simulink model "MicroFSMPCCLACPU1"  (R2024a)
settings: Solver=FixedStepAuto  StartTime=0.0  StopTime=Inf  RelTol=1e-3  EnableMultiTasking=on
values from neighbouring files (symbols this model uses):
  ar = single(round(1/10,3))    [Para_Motor_Micro.m]
  PI_params = mcb.internal.SetControllerParameters(pmsm,inverter,SI_System,T_pwm,Ts,Ts_speed)    [Para_Motor_Micro.m]
  Tabf = round(Tab',3)    [Para_Motor_Micro.m]
  target = mcb_SetProcessorDetails('F28379D',PWM_frequency)    [Para_Motor_Micro.m]
  Ts = T_pwm    (= 3e-05)    [Para_Motor_Micro.m]
  Ts_com = 2*1*Ts    (= 6e-05)    [Para_Motor_Micro.m]
undefined symbols (not defined in the file or in its folder): C28x, codertarget, CPU1, CPU2, Down, dyV, gmax, GPTRIP1SEL, GPTRIP2SEL, inverter, Ls, PWM_Counter_PeriodVel, R, Tab, Tv, Tvz, TZ1, TZ2, ud, Up
libraries: mcbcontrolslib x28, c2802xlib x18, c2837xDlib x13, dsparch4 x6, eeTransforms x5, slpidlib x4, mcbpositiondecoderlib x3, simulink x2, c2806xlib x1, spsabctoAlphaBetaZeroLib x1, c280xlib x1, c2000lib x1
(part 5 of 8)

== matlab function MicroFSMPCCLACPU1/ADC-PWM /Control_System/Current and BEMF gen Trapezoidal/Current trajectory2 ==
  settings: updateMethod=DISCRETE
  data: torq input; Ia output; th input; Ib output; moder output; eab output; w input
function [Ia,Ib,moder,eab]       = fcn(torq,th,w)

Ip=single(torq);


%%%% wrap

%tre = single((1)*th);
Ke=single(0.3631);
 f = single(2*pi);
 tr =single( mod(th,f));
i_A = single(0); i_B = single(0); 
mode=single(0);
e_A = single(0); e_B = single(0); e_C =single(0);


%%%%%%%%%Hexagono
if(0<=tr && tr<=pi/3)
    i_A = single(-3*tr*sqrt(3)/(2*pi));
     i_B = single(-3*tr/(2*pi) +1);

       elseif(pi/3<tr && tr<2*pi/3)
    i_A = single(-sqrt(3)/(2));
     i_B = single(-3*tr/(pi)+1.5);

       elseif(2*pi/3<tr && tr<pi)
    i_A =single( 3*tr*sqrt(3)/(2*pi)-3*sqrt(3)/(2));
     i_B = single(-3*tr/(2*pi) +1/2);

       elseif(pi<tr && tr<4*pi/3)
    i_A =single( 3*tr*sqrt(3)/(2*pi)-3*sqrt(3)/(2));
     i_B = single(3*tr/(2*pi) -5/2);

        elseif(4*pi/3<tr && tr<5*pi/3)
      i_A = single(sqrt(3)/(2));
     i_B =single( 3*tr/(pi)-4.5);

        elseif(5*pi/3<tr && tr<6*pi/3)
          i_A =single( -3*tr*sqrt(3)/(2*pi)+3*sqrt(3));
     i_B = single(3*tr/(2*pi) -2);
 
else
         i_A = single(0);
end



%%%%%%%%%FCEM%%%%%%%%%%%%
%% e_A
if(0<=tr && tr<=pi/6)
    e_A = single(6*tr/pi);
elseif((pi)/6<tr && tr<=5*pi/6)
    e_A = single(1);
  elseif(5*pi/6<tr && tr<=(7*pi)/6)
        e_A = single(-6*(tr-pi)/pi);
    elseif((7*pi)/6<tr && tr<11*pi/6)
        e_A = single(-1);
          elseif((11*pi)/6<tr && tr<12*pi/6)
        e_A =single(6*(tr-2*pi)/pi);
end
%% e_B
if(0<=tr && tr<=pi/2)
    e_B = single(-1);
elseif(pi/2<tr && tr<=(5*pi)/6)
    e_B =single( 6*(tr-4*pi/6)/pi);
elseif((5*pi)/6<tr && tr<=(3*pi)/2)
    e_B = single(1);
  elseif((3*pi)/2<tr && tr<=(11*pi)/6)
        e_B = single(-6*(tr-10*pi/6)/pi);
    elseif((11*pi)/6<tr && tr<2*pi)
        e_B = single(-1);
end
%% e_C
if(0<=tr && tr<=pi/6)
    e_C = single(1);
elseif(pi/6<tr && tr<=(pi)/2)
    e_C = single(-6*(tr-2*pi/6)/pi);
elseif((pi)/2<tr && tr<=(7*pi)/6)
    e_C = single(-1);
  elseif((7*pi)/6<tr && tr<=(3*pi)/2)
        e_C = single(6*(tr-8*pi/6)/pi);
    elseif((3*pi)/2<tr && tr<2*pi)
        e_C = single(1);
end



%%%%%
era=single(Ke*w*e_A);
erb=single(Ke*w*e_B);
erc=single(Ke*w*e_C);
%Ia=Ira;
ea=single((2/3)*(era-(1/2)*(erb)-(1/2)*erc));
eb=single((2/3)*((sqrt(3)/2)*(erb)-(sqrt(3)/2)*erc));

eab=[ea;eb];

%%%%%%%%%%%%%%%%%%%%%%%%

%%%%%%%%Moder%%%%%%%%%%%
if(0<=tr && tr<pi/6)
    mode=single(2);
elseif(pi/6<=tr && tr<(3*pi)/6)
      mode=single(3);
elseif((3*pi)/6<=tr && tr<(5*pi)/6)
    mode=single(4);
  elseif((5*pi)/6<=tr && tr<(7*pi)/6)
          mode=single(5);
    elseif((7*pi)/6<=tr && tr<(9*pi)/6)
         mode=single(6);     
    elseif((9*pi)/6<=tr && tr<(11*pi)/6)
        mode=single(1);
        elseif((11*pi)/6<=tr && tr<(12*pi)/6)
        mode=single(2);
end



moder=single(mode);
%%%%%%%%%%%%%%%%%%


Ia=Ip*2/sqrt(3)*i_A;
Ib=Ip*2/sqrt(3)*i_B;

%%%%%

== matlab function MicroFSMPCCLACPU1/ADC-PWM /Mesurments/Voltage Mesurment/Pole to phase 1 ==
  data: Vag input; Vn output; Vbg input; Vcg input

function Vn  = fcn(Vag,Vbg,Vcg)
% Vg=[Vag;Vbg;Vcg];
% Vn=[2/3,-1/3,-1/3;-1/3,2/3,-1/3;-1/3,-1/3,2/3]*Vg;
% 
 Van=single(2/3*Vag-1/3*Vbg -1/3*Vcg) ;
 Vbn=single(2/3*Vbg-1/3*Vag -1/3*Vcg) ;
 Vcn=single(2/3*Vcg-1/3*Vbg -1/3*Vag) ;
Vn=[Van;Vbn;Vcn];
end

== matlab function MicroFSMPCCLACPU1/ADC-PWM /Control_System/Current and BEMF gen Sinusoidal/Current trajectory1 ==
  settings: updateMethod=DISCRETE
  data: torq input; Ip output; th input; tr output; moder output
function [Ip,tr,moder]       = fcn(torq,th)
%Kt =0.3811;
%Kt=0.3455;
%J= 0.0002618;

%Ke=0.3739;
%Ke=single(0.3631);
%J=single(2.3998e-4);%%%Solo motor
%Ip=single((torq)/(2*Ke));
Ip=single((torq));
% the = (8/2)*th ;
 f = single(2*pi);
 tr =single( mod(th,f));
%tr = single((1)*th);

mode=single(0);


if(0<=tr && tr<pi/6)
    mode=single(2);
elseif(pi/6<=tr && tr<(3*pi)/6)
      mode=single(3);
elseif((3*pi)/6<=tr && tr<(5*pi)/6)
    mode=single(4);
  elseif((5*pi)/6<=tr && tr<(7*pi)/6)
          mode=single(5);
    elseif((7*pi)/6<=tr && tr<(9*pi)/6)
         mode=single(6);     
    elseif((9*pi)/6<=tr && tr<(11*pi)/6)
        mode=single(1);
        elseif((11*pi)/6<=tr && tr<(12*pi)/6)
        mode=single(2);
end




moder=single(mode);

== matlab function MicroFSMPCCLACPU1/ADC-PWM /Control_System/Closed Loop Control/Calculo directo BFEM1 ==
  settings: updateMethod=DISCRETE
  data: Iab input; u input; Iant input; FCEM output size=2
function FCEM     = fcn(Iab,u,Iant)

Ts=single(5e-05);
% R=single(1) ;
% L=single(2.002e-3);
R=single(1) ;
%L=single(9.75e-3);
 L=single(2.1e-3);
%M=(3/7)*L;
%Lt=(7/3)*M;
%Ls=single(L+M);
Ls=single(L);



ea=u(1)-(Ls/Ts)*Iab(1)-(R-(Ls/Ts))*Iant(1);
eb=u(2)-(Ls/Ts)*Iab(2)-(R-(Ls/Ts))*Iant(2);



FCEM=[ea;eb];

== matlab function MicroFSMPCCLACPU1/ADC-PWM /Control_System/Closed Loop Control/Clark Transform Filter/Calculo BEMF ==
  settings: updateMethod=DISCRETE
  data: I input; Iab output
function Iab            = fcn(I)



IA=I(1);
IB=I(2);
IC=I(3);

Ia=single((2/3)*(IA-(1/2)*(IB)-(1/2)*IC));
Ib=single((2/3)*((sqrt(3)/2)*(IB)-(sqrt(3)/2)*IC));

Iab=[Ia;Ib];





%%%%%

== matlab function MicroFSMPCCLACPU1/ADC-PWM /Control_System/CLA Subsystem Current control/Calculo directo BFEM1 ==
  settings: updateMethod=DISCRETE
  data: Iab input; u input; Iant input; FCEM output size=2
function FCEM     = fcn(Iab,u,Iant)

Ts=single(5e-05);
% R=single(1) ;
% L=single(2.002e-3);
R=single(1) ;
%L=single(9.75e-3);
 L=single(2.1e-3);
%M=(3/7)*L;
%Lt=(7/3)*M;
%Ls=single(L+M);
Ls=single(L);



ea=u(1)-(Ls/Ts)*Iab(1)-(R-(Ls/Ts))*Iant(1);
eb=u(2)-(Ls/Ts)*Iab(2)-(R-(Ls/Ts))*Iant(2);



FCEM=[ea;eb];

== matlab function MicroFSMPCCLACPU1/ADC-PWM /Control_System/Closed Loop Control/Current trajectory1 ==
  settings: updateMethod=DISCRETE
  data: torq input; Ia output; th input; Ib output; moder output
function [Ia,Ib,moder]       = fcn(torq,th)
%Kt =0.3811;
%Kt=0.3455;
%J= 0.0002618;
%Ip=single((torq)/(2*Kt));
Ip=single(torq);
% p=single(8);
% Am =single( (6/pi));
% mph = single(pi/3);
%%%% wrap
tr = single((1)*th);
 %f = single(2*pi);
%tr =single( mod(the,f));
i_A = single(0); i_B = single(0); i_C =single(0);
mode=single(0);


%%%%%%%%%Hexagono
% if(0<=tr && tr<=pi/3)
%     i_A = single(0);
%      i_B = single(2/(sqrt(3)));
% 
%        elseif(pi/3<tr && tr<2*pi/3)
%     i_A = single(-1);
%      i_B = single(1/(sqrt(3)));
% 
%        elseif(2*pi/3<tr && tr<pi)
%     i_A =single(-1);
%      i_B = single(-1/(sqrt(3)));
% 
%        elseif(pi<tr && tr<4*pi/3)
%     i_A =single(0);
%      i_B = single(-2/(sqrt(3)));
% 
%         elseif(4*pi/3<tr && tr<5*pi/3)
%       i_A = single(1);
%      i_B =single( -1/(sqrt(3)));
% 
%         elseif(5*pi/3<tr && tr<6*pi/3)
%           i_A =single( 1);
%      i_B = single(3*tr/(2*pi) -2);
%  
% else
%          i_A = single(0);
% end


%%%%%%%%%%%%%%%%%%
if(0<=tr && tr<pi/6)
    mode=single(2);
      i_A = single(0);
     i_B = single(2/(sqrt(3)));

elseif(pi/6<=tr && tr<(3*pi)/6)
      mode=single(3);
         i_A = single(-1);
     i_B = single(1/(sqrt(3)));

elseif((3*pi)/6<=tr && tr<(5*pi)/6)
    mode=single(4);
    i_A =single(-1);
     i_B = single(-1/(sqrt(3)));

  elseif((5*pi)/6<=tr && tr<(7*pi)/6)
          mode=single(5);
              i_A =single(0);
     i_B = single(-2/(sqrt(3)));

    elseif((7*pi)/6<=tr && tr<(9*pi)/6)
         mode=single(6);     
            i_A =single(1);
            i_B = single(-1/(sqrt(3)));
  
    elseif((9*pi)/6<=tr && tr<(11*pi)/6)
        mode=single(1);
                i_A =single( 1);
     i_B = single(1/(sqrt(3)));
        elseif((11*pi)/6<=tr && tr<(12*pi)/6)
        mode=single(2);
     i_A = single(0);
     i_B = single(2/(sqrt(3)));
end
moder=single(mode);



Ia=Ip*i_A;
Ib=Ip*i_B;

%%%%%

== matlab function MicroFSMPCCLACPU1/ADC-PWM /Control_System/Closed Loop Control/Current trajectory12 ==
  settings: updateMethod=DISCRETE
  data: torq input; Ia output; th input; Ib output; mod12 output single size=1; mod6 output single size=1
function [Ia,Ib,mod12,mod6]       = fcn(torq,th)
%Kt =0.3811;
%Kt=0.3455;
%J= 0.0002618;
%Ip=single((torq)/(2*Kt));
Ip=single(torq);
% p=single(8);
% Am =single( (6/pi));
% mph = single(pi/3);
%%%% wrap
tr = single((1)*th);
 %f = single(2*pi);
%tr =single( mod(the,f));
i_A = single(0); i_B = single(0); i_C =single(0);
mode1=single(0);
mode=single(0);

%%%% e_A

if(0<=tr && tr<=pi/6)
    i_A = single(0);
elseif((pi)/6<tr && tr<=5*pi/6)
    i_A = single(-1);
  elseif(5*pi/6<tr && tr<=(7*pi)/6)
        i_A =single( 0);
    elseif((7*pi)/6<tr && tr<11*pi/6)
        i_A = single(1);
          elseif((11*pi)/6<tr && tr<12*pi/6)
        i_A =single(0);
end
%%%% i_B
if(0<=tr && tr<=pi/2)
    i_B = single(1);
elseif(pi/2<tr && tr<=(5*pi)/6)
    i_B = single(0);
elseif((5*pi)/6<tr && tr<=(3*pi)/2)
    i_B = single(-1);
  elseif((3*pi)/2<tr && tr<=(11*pi)/6)
        i_B =single(0);
    elseif((11*pi)/6<tr && tr<2*pi)
        i_B = single(1);
end
%%%% i_C
if(0<=tr && tr<=pi/6)
    i_C = single(-1);
elseif(pi/6<tr && tr<=(pi)/2)
    i_C =single( 0);
elseif((pi)/2<tr && tr<=(7*pi)/6)
    i_C = single(1);
  elseif((7*pi)/6<tr && tr<=(3*pi)/2)
        i_C = single(0);
    elseif((3*pi)/2<tr && tr<2*pi)
        i_C = single(-1);
end
%%%mode
% 
% if(0<=tr && tr<pi/3)
%     mode=1;
% elseif(pi/3<=tr && tr<(2*pi)/3)
%       mode=2;
% elseif((2*pi)/3<=tr && tr<pi)
%     mode=3;
%   elseif(pi<=tr && tr<(4*pi)/3)
%           mode=4;
%     elseif((4*pi)/3<=tr && tr<(5*pi)/3)
%          mode=5;     
%     elseif((5*pi)/3<=tr && tr<2*pi)
%         mode=6;
% end
% 

% if(0<=tr && tr<pi/3)
%     mode=single(1);
% elseif(pi/3<=tr && tr<(2*pi)/3)
%       mode=single(2);
% elseif((2*pi)/3<=tr && tr<pi)
%     mode=single(3);
%   elseif(pi<=tr && tr<(4*pi)/3)
%           mode=single(4);
%     elseif((4*pi)/3<=tr && tr<(5*pi)/3)
%          mode=single(5);     
%     elseif((5*pi)/3<=tr && tr<(6*pi)/3)
%         mode=single(6);
%  end
% moder=single(mode);


% if(0<=tr && tr<pi/6)
%     mode1=single(2);
% elseif(pi/6<=tr && tr<(3*pi)/6)
%       mode1=single(3);
% elseif((3*pi)/6<=tr && tr<(5*pi)/6)
%     mode1=single(4);
%   elseif((5*pi)/6<=tr && tr<(7*pi)/6)
%           mode1=single(5);
%     elseif((7*pi)/6<=tr && tr<(9*pi)/6)
%          mode1=single(6);     
%     elseif((9*pi)/6<=tr && tr<(11*pi)/6)
%         mode1=single(1);
%         elseif((11*pi)/6<=tr && tr<(12*pi)/6)
%         mode1=single(2);
% end



% %%%%12%%%
if(0<=tr && tr<pi/6)
    mode=single(4);
    mode1=single(2);
elseif(pi/6<=tr && tr<(2*pi)/6)
      mode=single(5);
         mode1=single(3);
elseif(2*pi/6<=tr && tr<(3*pi)/6)
      mode=single(6);
         mode1=single(3);
elseif((3*pi)/6<=tr && tr<(4*pi)/6)
    mode=single(7);
    mode1=single(4);
elseif((4*pi)/6<=tr && tr<(5*pi)/6)
    mode=single(8); 
     mode1=single(4);
 elseif((5*pi)/6<=tr && tr<(6*pi)/6)
          mode=single(9);
           mode1=single(5);
 elseif((6*pi)/6<=tr && tr<(7*pi)/6)
          mode=single(10);   
                   mode1=single(5);
    elseif((7*pi)/6<=tr && tr<(8*pi)/6)
         mode=single(11); 
                  mode1=single(6);
  elseif((8*pi)/6<=tr && tr<(9*pi)/6)
         mode=single(12);      
          mode1=single(6);
    elseif((9*pi)/6<=tr && tr<(10*pi)/6)
        mode=single(1);
         mode1=single(1);
    elseif((10*pi)/6<=tr && tr<(11*pi)/6)
        mode=single(2);
            mode1=single(1);
        elseif((11*pi)/6<=tr && tr<(12*pi)/6)
        mode=single(3);
        mode1=single(2);
end

%%%%%



mod6=single(mode1);
mod12=single(mode);
%%%%%
Ira=single(Ip*i_A);
Irb=single(Ip*i_B);
Irc=single(Ip*i_C);
%Ia=Ira;
Ia=single((2/3)*(Ira-(1/2)*(Irb)-(1/2)*Irc));
Ib=single((2/3)*((sqrt(3)/2)*(Irb)-(sqrt(3)/2)*Irc));

%%%%%

== matlab function MicroFSMPCCLACPU1/ADC-PWM /Control_System/Closed Loop Control/Current trayectory moder12 ==
  settings: updateMethod=DISCRETE
  data: torq input; Ia output; th input; Ib output; selector output; moder output
function [Ia,Ib,selector,moder]       = fcn(torq,th)
%Kt =0.3811;
% Kt=0.3739;
% J= 2.9795e-04;
%Ip=(J*torq)/(2*Kt);
Ip=single(torq);
p=single(8);
Am =single( (6/pi));
mph = single(pi/3);
%%%% wrap
tr = single((1)*th);
%tr2 = mod(the,f);
trb=tr-(2*pi)/3;
if (trb<0)
  trb=trb+2*pi;  
end
trc=tr-(4*pi)/3;
if (trc<0)
  trc=trc+2*pi;  
end
i_A =single( 0); i_B = single( 0); i_C = single( 0);
mode=single(0);
mode1=single(0);
%%%% e_A
%%%%%%Hexagono%%%%%
if(0<=tr && tr<=pi/3)
    i_A = single(-3*tr*sqrt(3)/(2*pi));
     i_B = single(-3*tr/(2*pi) +1);

       elseif(pi/3<tr && tr<2*pi/3)
    i_A = single(-sqrt(3)/(2));
     i_B = single(-3*tr/(pi)+1.5);

       elseif(2*pi/3<tr && tr<pi)
    i_A = single(3*tr*sqrt(3)/(2*pi)-3*sqrt(3)/(2));
     i_B = single(-3*tr/(2*pi) +1/2);

       elseif(pi<tr && tr<4*pi/3)
    i_A =single( 3*tr*sqrt(3)/(2*pi)-3*sqrt(3)/(2));
     i_B =single( 3*tr/(2*pi) -5/2);

        elseif(4*pi/3<tr && tr<5*pi/3)
      i_A =single( sqrt(3)/(2));
     i_B = single(3*tr/(pi)-4.5);

        elseif(5*pi/3<tr && tr<6*pi/3)
          i_A =single( -3*tr*sqrt(3)/(2*pi)+3*sqrt(3));
     i_B = single(3*tr/(2*pi) -2);
 
else
         i_A = single(0);
end
%%%%%%%%%%%%%%%%%%%%%%%
%%%%%%%Normal
%%%% e_A

% if(0<=tr && tr<=pi/6)
%     i_A =0;
% elseif((pi)/6<tr && tr<=5*pi/6)
%     i_A = -1;
%   elseif(5*pi/6<tr && tr<=(7*pi)/6)
%         i_A =0;
%     elseif((7*pi)/6<tr && tr<11*pi/6)
%         i_A = 1;
%           elseif((11*pi)/6<tr && tr<12*pi/6)
%         i_A =0;
% end
% %%%% i_B
% if(0<=tr && tr<=pi/2)
%     i_B = 1;
% elseif(pi/2<tr && tr<=(5*pi)/6)
%     i_B = 0;
% elseif((5*pi)/6<tr && tr<=(3*pi)/2)
%     i_B = -1;
%   elseif((3*pi)/2<tr && tr<=(11*pi)/6)
%         i_B =0;
%     elseif((11*pi)/6<tr && tr<2*pi)
%         i_B = 1;
% end
% %%%% i_C
% if(0<=tr && tr<=pi/6)
%     i_C = -1;
% elseif(pi/6<tr && tr<=(pi)/2)
%     i_C =0;
% elseif((pi)/2<tr && tr<=(7*pi)/6)
%     i_C = 1;
%   elseif((7*pi)/6<tr && tr<=(3*pi)/2)
%         i_C = 0;
%     elseif((3*pi)/2<tr && tr<2*pi)
%         i_C = -1;
% end
%%%%%%%%%%

%%%mode
% 
% if(0<=tr && tr<pi/3)
%     mode=1;
% elseif(pi/3<=tr && tr<(2*pi)/3)
%       mode=2;
% elseif((2*pi)/3<=tr && tr<pi)
%     mode=3;
%   elseif(pi<=tr && tr<(4*pi)/3)
%           mode=4;
%     elseif((4*pi)/3<=tr && tr<(5*pi)/3)
%          mode=5;     
%     elseif((5*pi)/3<=tr && tr<2*pi)
%         mode=6;
% end
% 
% if(0<=tr && tr<pi/6)
%     mode=2;
% elseif(pi/6<=tr && tr<(3*pi)/6)
%       mode=3;
% elseif((3*pi)/6<=tr && tr<(5*pi)/6)
%     mode=4;
%   elseif((5*pi)/6<=tr && tr<(7*pi)/6)
%           mode=5;
%     elseif((7*pi)/6<=tr && tr<(9*pi)/6)
%          mode=6;     
%     elseif((9*pi)/6<=tr && tr<(11*pi)/6)
%         mode=1;
%         elseif((11*pi)/6<=tr && tr<(12*pi)/6)
%         mode=2;
% end
% moder=mode;

if(0<=tr && tr<pi/6)
    mode1=single(2);
elseif(pi/6<=tr && tr<(3*pi)/6)
      mode1=single(3);
elseif((3*pi)/6<=tr && tr<(5*pi)/6)
    mode1=single(4);
  elseif((5*pi)/6<=tr && tr<(7*pi)/6)
          mode1=single(5);
    elseif((7*pi)/6<=tr && tr<(9*pi)/6)
         mode1=single(6);     
    elseif((9*pi)/6<=tr && tr<(11*pi)/6)
        mode1=single(1);
        elseif((11*pi)/6<=tr && tr<(12*pi)/6)
        mode1=single(2);
end


%%%%24%%%
% if(0<=tr && tr<pi/12)
%     mode=7;
%     elseif(pi/12<=tr && tr<(2*pi)/12)
%       mode=8;
%      elseif(2*pi/12<=tr && tr<(3*pi)/12)
%       mode=9;
%      elseif(3*pi/12<=tr && tr<(4*pi)/12)
%       mode=10;
%         elseif(4*pi/12<=tr && tr<(5*pi)/12)
%       mode=11;
%         elseif(5*pi/12<=tr && tr<(6*pi)/12)
%       mode=12;
%         elseif(6*pi/12<=tr && tr<(7*pi)/12)
%       mode=13;
%         elseif(7*pi/12<=tr && tr<(8*pi)/12)
%       mode=14;
%         elseif(8*pi/12<=tr && tr<(9*pi)/12)
%       mode=15;
%          elseif(9*pi/12<=tr && tr<(10*pi)/12)
%       mode=16;
%            elseif(10*pi/12<=tr && tr<(11*pi)/12)
%       mode=17;
%            elseif(11*pi/12<=tr && tr<(12*pi)/12)
%       mode=18;
%            elseif(12*pi/12<=tr && tr<(13*pi)/12)
%       mode=19;
%            elseif(13*pi/12<=tr && tr<(14*pi)/12)
%       mode=20;
%            elseif(14*pi/12<=tr && tr<(15*pi)/12)
%       mode=21;
%            elseif(15*pi/12<=tr && tr<(16*pi)/12)
%       mode=22;
%            elseif(16*pi/12<=tr && tr<(17*pi)/12)
%       mode=23;
%            elseif(17*pi/12<=tr && tr<(18*pi)/12)
%       mode=24;  
%        
%           elseif((9*pi)/6<=tr && tr<(19*pi)/12)
%         mode=1;
%     elseif((19*pi)/12<=tr && tr<(20*pi)/12)
%         mode=2;
%         elseif((20*pi)/12<=tr && tr<(21*pi)/12)
%         mode=3;
%          elseif((21*pi)/12<=tr && tr<(22*pi)/12)
%         mode=4;
%           elseif((22*pi)/12<=tr && tr<(23*pi)/12)
%         mode=5;
%             elseif((23*pi)/12<=tr && tr<(24*pi)/12)
%         mode=6;
% end

%%%%%




% %%%%12%%%
if(0<=tr && tr<pi/6)
    mode=single(4);
elseif(pi/6<=tr && tr<(2*pi)/6)
      mode=single(5);
elseif(2*pi/6<=tr && tr<(3*pi)/6)
      mode=single(6);
elseif((3*pi)/6<=tr && tr<(4*pi)/6)
    mode=single(7);
elseif((4*pi)/6<=tr && tr<(5*pi)/6)
    mode=single(8);    
 elseif((5*pi)/6<=tr && tr<(6*pi)/6)
          mode=single(9);
 elseif((6*pi)/6<=tr && tr<(7*pi)/6)
          mode=single(10);        
    elseif((7*pi)/6<=tr && tr<(8*pi)/6)
         mode=single(11); 
  elseif((8*pi)/6<=tr && tr<(9*pi)/6)
         mode=single(12);         
    elseif((9*pi)/6<=tr && tr<(10*pi)/6)
        mode=single(1);
    elseif((10*pi)/6<=tr && tr<(11*pi)/6)
        mode=single(2);
        elseif((11*pi)/6<=tr && tr<(12*pi)/6)
        mode=single(3);
end

%%%%%


 moder=mode1;
 selector=mode;
%%%%%
Ira=Ip*i_A;
Irb=Ip*i_B;
Irc=Ip*i_C;
%Ia=Ira;
% Ia=(2/3)*(Ira-(1/2)*(Irb)-(1/2)*Irc);
% Ib=(2/3)*((sqrt(3)/2)*(Irb)-(sqrt(3)/2)*Irc);
Ia=Ip*2/sqrt(3)*i_A;
Ib=Ip*2/sqrt(3)*i_B;
%%%%%

== matlab function MicroFSMPCCLACPU1/ADC-PWM /Control_System/Closed Loop Control/FS-MPC 2 Vectores correcion moder ==
  settings: updateMethod=DISCRETE
  data: I input; Gate output size=3; FEM input; iAref input; iBref input; J output size=1; Vbus input; Vpred output; mode input; Ipred output

function [Gate,J,Vpred,Ipred]      = fcn(I,FEM,iAref,iBref,Vbus,mode)


%%%%%Init Parameters%%%%%%%
Ts=single(5e-5);
R=single(1.2) ;
L=single(4.75e-3);
M=L;
Lt=(7/3)*M;
Ls=single(Lt+M);
%ud=240;
ud=single(170);
Kt =single(0.3811);
%T0=Ts*(1);
Ke=single(0.3455);
gmax=single(100000);
n=single(3);
Tp=single(Ts*0.9);
uAnull=single(0);
uBnull=single(0);
 persistent    Gop jop Gates iApred iBpred %status1 %tick status1 
     if isempty(Gates)
        Gates=[0,0,0]';
        Gop=gmax;
        jop=single(1);
        iApred=single(0);
        iBpred=single(0);
% status1=[0,0,0;
%  1,0,0	;
% 1,1,0;]; 
     end


%%%%%%Read mesurments%%%%%%%%%%%%
iA=I(1);
iB=I(2);
eA=FEM(1);
eB=FEM(2);
% eA1=FEM1(1);
% eB1=FEM1(2);
% fa=eA/(Ke*w);
% fb=eB/(Ke*w);
% fa1=fa;
% fb1=fb;
% ua=u(1);
% ub=u(2);



 % % %%%7 vectores ordenados ab separados flotando
%  status1=[0,1,0,1,0,1	;
%      1,0,0,0,0,1	;
%  0,0,1,0,0,1	;
%  0,1,1,0,0,0	;
%  0,1,0,0,1,0	;
%  0,0,0,1,1,0	;
%  1,0,0,1,0,0	;];
% 
%  u1=ud*[0	,	0	;
%      1/2	,	sqrt(3)/6 	;
% 0	,	sqrt(3)/3	;
% -1/2	,	sqrt(3)/6 	;
% -1/2	,	-sqrt(3)/6 	;
% 0	,	-sqrt(3)/3	;
% 1/2	,	-sqrt(3)/6 	;
% ];

%%%%%%For loop 3%%%%%%      
% %%%7 vectores ordenados ab tradicionales
%  status1=[1,1,1;
%           1,0,0	;
%           1,1,0;
%           0,1,0;
%            0,1,1	;
%            0,0,1	;
%            1,0,1;
%            ];
% % 
%  u1=ud*[0	,	0	;
%       2/3	,	0	;
%       1/3	,	1/sqrt(3)	;%parece estar aml el vector
%   -1/3	,	1/sqrt(3)	;
%  -2/3	,	0	;
%  -1/3	,	-1/sqrt(3)	;
%   1/3	,	-1/sqrt(3)	;
%   ];

%%%%%Modos 2 vectores con VO

 if mode==1
 status1=[0,0,0;
 1,0,0	;
1,1,0;];   
 u1=ud*[0	,	0	;
2/3	,	0	;
1/3	,	1/sqrt(3)];
elseif mode==2
 status1=[0,0,0;
1,1,0	;
0,1,0	;];   
 u1=ud*[0	,	0	;
1/3	,	1/sqrt(3)	;
-1/3	,	1/sqrt(3)	;];   
elseif mode==3
 status1=[0,0,0;
0,1,0	;
0,1,1	;];   
 u1=ud*[0	,	0	;
-1/3	,	1/sqrt(3)	;
-2/3	,	0	;];  
 elseif mode==4
 status1=[0,0,0;
 0,1,1	;
0,0,1	;];   
 u1=ud*[0	,	0	;
-2/3	,	0	;
-1/3	,	-1/sqrt(3)	;];
 elseif mode==5
 status1=[0,0,0;
 0,0,1	;
1,0,1	;];   
 u1=ud*[0	,	0	;
-1/3	,	-1/sqrt(3)	;
1/3	,	-1/sqrt(3)	;];
 elseif mode==6
 status1=[0,0,0
1,0,1	;
 1,0,0	;];   
 u1=ud*[0	,	0	;
1/3	,	-1/sqrt(3)	;
2/3	,	0	;];

else
 status1=[0,0,0;
 1,0,0	;
1,1,0;];   
 u1=ud*[0	,	0	;
2/3	,	0	;
1/3	,	1/sqrt(3)]; 
end


%%%%%%%%FSMPC%%%%%%%%%%%%%%%%%%%%%%%%%%%%%%%%%%%%%

     Gop=gmax;
      jop=single(1);

%%%%%%For n loop  %%%%%% 
     for j= 1:n    
     uA1=u1(j,1);
     uB1=u1(j,2);

     iA1= iA + (1/Ls)*(Tp*uA1)- (Ts/Ls)*(eA+R*iA);
     iB1=iB + (1/Ls)*(Tp*uB1)- (Ts/Ls)*(eB+R*iB);
     
     G=abs(iAref-iA1)+abs(iBref-iB1) ; 

          if G<Gop
          Gop=G;
          jop=j;
          iApred=iA1;
          iBpred=iB1;
          end
     end

    
%%%%Apply conmutation states%%%%%%%%%%%%%%%%%%%%%%%  

    Gates=status1(jop,:)';
UA=Tp/Ts*u1(jop,1) ;%+(Ts-Tp)/Ts*uAnull;
UB=Tp/Ts*u1(jop,2) ;%+(Ts-Tp)/Ts*uBnull;
%Gates=status1(jop,:)';
J=jop;
Gate=Gates;
Vpred=[UA;UB];
Ipred=[iApred;iBpred];
%tie=t2;
%jl=jn;
%j=1;

== matlab function MicroFSMPCCLACPU1/ADC-PWM /Control_System/Closed Loop Control/FS-MPC 2 Vectores modulado ==
  settings: updateMethod=DISCRETE
  data: I input; Gate output size=3; FEM input size=2; iAref input; iBref input; J output size=1; Vbus input; Vpred output; mode input; Ipred output

function [Gate,J,Vpred,Ipred]      = fcn(I,FEM,iAref,iBref,Vbus,mode)


%%%%%Init Parameters%%%%%%%
Ts=single(5e-05);
R=single(1.2) ;
L=single(4.75e-3);
M=L;
Lt=(7/3)*M;
Ls=single(Lt+M);
%ud=240;
ud=single(170);
Kt =single(0.3811);
%T0=Ts*(1);
Ke=single(0.3455);
gmax=single(100000);
n=single(15);

uAnull=single(0);
uBnull=single(0);
Div=single(4); %%%%Numero de divisiones 
dy0=single(0.1);
dyV=(1-dy0)/Div;


%Tp=single(Ts*0.9);
 persistent    Gop jop Gates iApred iBpred  uApred uBpred status1 %tick status1 
     if isempty(Gates)
        Gates=single([0,0,0]');
        Gop=gmax;
        jop=single(1);
        iApred=single(0);
        iBpred=single(0);
        uApred=single(0);
        uBpred=single(0);
        status1=[0,0,0;
 1,1,0;
 0,1,0;]; 
     end


%%%%%%Read mesurments%%%%%%%%%%%%
iA=I(1);
iB=I(2);
eA=FEM(1);
eB=FEM(2);
moder=mode;
% eA1=FEM1(1);
% eB1=FEM1(2);
% fa=eA/(Ke*w);
% fb=eB/(Ke*w);
% fa1=fa;
% fb1=fb;
% ua=u(1);
% ub=u(2);



 % % %%%7 vectores ordenados ab separados flotando
%  status1=[0,1,0,1,0,1	;
%      1,0,0,0,0,1	;
%  0,0,1,0,0,1	;
%  0,1,1,0,0,0	;
%  0,1,0,0,1,0	;
%  0,0,0,1,1,0	;
%  1,0,0,1,0,0	;];
% 
%  u1=ud*[0	,	0	;
%      1/2	,	sqrt(3)/6 	;
% 0	,	sqrt(3)/3	;
% -1/2	,	sqrt(3)/6 	;
% -1/2	,	-sqrt(3)/6 	;
% 0	,	-sqrt(3)/3	;
% 1/2	,	-sqrt(3)/6 	;
% ];

%%%%%%For loop 3%%%%%%      
% %%%7 vectores ordenados ab tradicionales
%  status1=[1,1,1;
%           1,0,0	;
%           1,1,0;
%           0,1,0;
%            0,1,1	;
%            0,0,1	;
%            1,0,1;
%            ];
% % 
%  u1=ud*[0	,	0	;
%       2/3	,	0	;
%       1/3	,	1/sqrt(3)	;%parece estar aml el vector
%   -1/3	,	1/sqrt(3)	;
%  -2/3	,	0	;
%  -1/3	,	-1/sqrt(3)	;
%   1/3	,	-1/sqrt(3)	;
%   ];
indexv=[1,1,1,1,1,1,1,1,1,1,2,2,2,2,3;
        1,1,1,1,1,1,2,2,2,3,2,2,2,3,3;
        1,1,1,2,2,3,2,2,3,3,2,2,3,3,3;
        1,2,3,2,3,3,2,3,3,3,2,3,3,3,3;];
%%%%%Modos 2 vectores con VO
if mode==1
 status1=[0,0,0;
1,1,0	;
0,1,0	;];   
 u1=ud*[0	,	0	;
1/3	,	1/sqrt(3)	;
-1/3	,	1/sqrt(3)	;];   
elseif mode==2
 status1=[0,0,0;
0,1,0	;
0,1,1	;];   
 u1=ud*[0	,	0	;
-1/3	,	1/sqrt(3)	;
-2/3	,	0	;];  
 elseif mode==3
 status1=[0,0,0;
 0,1,1	;
0,0,1	;];   
 u1=ud*[0	,	0	;
-2/3	,	0	;
-1/3	,	-1/sqrt(3)	;];
 elseif mode==4
 status1=[0,0,0;
 0,0,1	;
1,0,1	;];   
 u1=ud*[0	,	0	;
-1/3	,	-1/sqrt(3)	;
1/3	,	-1/sqrt(3)	;];
 elseif mode==5
 status1=[0,0,0
1,0,1	;
 1,0,0	;];   
 u1=ud*[0	,	0	;
1/3	,	-1/sqrt(3)	;
2/3	,	0	;];
 elseif mode==6
 status1=[0,0,0;
 1,0,0	;
1,1,0;];   
 u1=ud*[0	,	0	;
2/3	,	0	;
1/3	,	1/3	;];
else
   status1=[0,0,0;
1,1,0	;
0,1,0	;];   
 u1=ud*[0	,	0	;
1/3	,	1/sqrt(3)	;
-1/3	,	1/sqrt(3)	;]; 
end

Vpred=[uApred;uBpred];

%%%%%%%%FSMPC%%%%%%%%%%%%%%%%%%%%%%%%%%%%%%%%%%%%%

     Gop=gmax;
      jop=single(1);

%%%%%%For n loop  %%%%%% 
     for j= 1:n    
     uA1=u1(indexv(1,j),1);
     uB1=u1(indexv(1,j),2);
     uA2=u1(indexv(2,j),1);
     uB2=u1(indexv(2,j),2);
     uA3=u1(indexv(3,j),1);
     uB3=u1(indexv(3,j),2);
     uA4=u1(indexv(4,j),1);
     uB4=u1(indexv(4,j),2);

%%%%%%For loop 3 combinacion de vectores%%%%%% 

       uA=dyV*(uA1 + uA2+ uA3 + uA4)+dy0*uAnull;
       uB=dyV*(uB1 + uB2+ uB3 + uB4)+dy0*uAnull;


     iA1= iA + (1/Ls)*(Ts*uA)- (Ts/Ls)*(eA+R*iA);
     iB1=iB + (1/Ls)*(Ts*uB)- (Ts/Ls)*(eB+R*iB);
     
     G=(iAref-iA1)^2+(iBref-iB1)^2 ; 

          if G<Gop
          Gop=G;
          jop=j;
          iApred=iA1;
          iBpred=iB1;
          uApred=uA;
          uBpred=uB;
          end
     end

    
%%%%Apply conmutation states%%%%%%%%%%%%%%%%%%%%%%%  


   % Gates=status1(jop,:)';

To=dyV*((indexv(1,jop)==1)+(indexv(2,jop)==1)+(indexv(3,jop)==1)+(indexv(4,jop)==1))+dy0;
Ta=dyV*((indexv(1,jop)==2)+(indexv(2,jop)==2)+(indexv(3,jop)==2)+(indexv(4,jop)==2));
Tb=dyV*((indexv(1,jop)==3)+(indexv(2,jop)==3)+(indexv(3,jop)==3)+(indexv(4,jop)==3));


TA=(moder==6)*(To+Tb+Ta)+(moder==5)*(To+Tb+Ta)+(moder==1)*(To+Ta)+(moder==2)*(To)+(moder==3)*(To)+(moder==4)*(To+Tb);
TB=(moder==5)*(To)+(moder==6)*(To+Tb)+(moder==1)*(To+Tb+Ta)+(moder==2)*(To+Tb+Ta)+(moder==3)*(To+Ta)+(moder==4)*(To);
TC=(moder==5)*(To+Ta)+(moder==6)*(To)+(moder==1)*(To)+(moder==2)*(To+Tb)+(moder==3)*(To+Tb+Ta)+(moder==4)*(To+Tb+Ta);

Gates=[TA,TB,TC]';
J=jop;
Gate=Gates;
Ipred=[iApred;iBpred];
%tie=t2;
%jl=jn;
%j=1;

== matlab function MicroFSMPCCLACPU1/ADC-PWM /Control_System/Closed Loop Control/FS-MPC 2 Vectores modulado Clean ==
  settings: updateMethod=DISCRETE
  data: I input; Gate output size=3; FEM input size=2; iAref input; iBref input; mode input; Ts parameter; R parameter; Ls parameter; ud parameter; gmax parameter; dyV parameter; Tab parameter

function Gate       = fcn(I,FEM,iAref,iBref,mode,Ts, R, Ls, ud, gmax,dyV, Tab)


%%%%%Init Parameters%%%%%%%

% Ts=single(2.5e-5);
% R=single(1) ;
%  L=single(2.02e-3);
%  M=(3/7)*L;
% %Lt=(7/3)*M;
% Ls=single(L+M);
% ud=single(170);
% gmax=single(1000);
n=single(15);

% Div=single(4); %%%%Numero de divisiones 
% dy0=single(0.12);
% dyV=(1-dy0);


%Tp=single(Ts*0.9);
 persistent    Gop jop Gates iApred iBpred  uApred uBpred status1 %tick status1 
     if isempty(Gates)
        Gates=single([0,0,0]');
        Gop=gmax;
        jop=single(1);
        iApred=single(0);
        iBpred=single(0);
        uApred=single(0);
        uBpred=single(0);
  
     end


%%%%%%Read mesurments%%%%%%%%%%%%
iA=I(1);
iB=I(2);
eA=FEM(1);
eB=FEM(2);
moder=mode;

% % 
% % indexv=[1,1,1,1,1,1,1,1,1,1,2,2,2,2,3;
% %         1,1,1,1,1,1,2,2,2,3,2,2,2,3,3;
% %         1,1,1,2,2,3,2,2,3,3,2,2,3,3,3;
% %         1,2,3,2,3,3,2,3,3,3,2,3,3,3,3;];

% Tab=[0 0;
%     0.25 0;
%     0 0.25;
%     0.5 0;
%     0.25 0.25
%     0 0.5;
%     0.75 0;
%     0.5 0.25;
%     0.25 0.5;
%     0 0.75;
%     1 0;
%     0.75 0.25
%     0.5 0.5
%     0.25 0.75
%     0 1];

if mode==1
   u1=ud*[0	,	0	;
2/3	,	0	;
1/3	,	1/sqrt(3)];
elseif mode==2
   u1=ud*[0	,	0	;
1/3	,	1/sqrt(3)	;
-1/3	,	1/sqrt(3)	;];   
elseif mode==3
   u1=ud*[0	,	0	;
-1/3	,	1/sqrt(3)	;
-2/3	,	0	;];  
 elseif mode==4
   u1=ud*[0	,	0	;
-2/3	,	0	;
-1/3	,	-1/sqrt(3)	;];
 elseif mode==5
   u1=ud*[0	,	0	;
-1/3	,	-1/sqrt(3)	;
1/3	,	-1/sqrt(3)	;];
 elseif mode==6
  u1=ud*[0	,	0	;
1/3	,	-1/sqrt(3)	;
2/3	,	0	;];
else
  u1=ud*[0	,	0	;
2/3	,	0	;
1/3	,	1/sqrt(3)]; 
end

%%%%%%%%FSMPC%%%%%%%%%%%%%%%%%%%%%%%%%%%%%%%%%%%%%

     Gop=gmax;
     jop=single(1);
     uA1=u1(2,1);
     uB1=u1(2,2);
     uA2=u1(3,1);
     uB2=u1(3,2);

%%%%%%For n loop  %%%%%% 
     for j= 1:n    
   
    T1=Tab(j,1);
    T2=Tab(j,2);
    uA=dyV*(T1*uA1 + T2*uA2);%+dy0*uAnull;
    uB=dyV*(T1*uB1 + T2*uB2);%+dy0*uAnull;

%%%%%%For loop 3 combinacion de vectores%%%%%% 

     iA1= iA + (1/Ls)*(Ts*uA)- (Ts/Ls)*(eA+R*iA);
     iB1=iB + (1/Ls)*(Ts*uB)- (Ts/Ls)*(eB+R*iB);
     
     G=(iAref-iA1)^2+(iBref-iB1)^2 ; 

          if G<Gop
          Gop=G;
          jop=j;
          
          end
     end
%%%%Apply conmutation states%%%%%%%%%%%%%%%%%%%%%%%  
Ta=dyV*Tab(jop,1);
Tb=dyV*Tab(jop,2);

TA=(moder==1)*(Tb+Ta)+(moder==6)*(Tb+Ta)+(moder==2)*(Ta)+(moder==5)*(Tb);
TB=(moder==1)*(Tb)+(moder==2)*(Tb+Ta)+(moder==3)*(Tb+Ta)+(moder==4)*(Ta);
TC=(moder==6)*(Ta)+(moder==3)*(Tb)+(moder==4)*(Tb+Ta)+(moder==5)*(Tb+Ta);
  

Gates=[TA,TB,TC]';
Gate=Gates;

== matlab function MicroFSMPCCLACPU1/ADC-PWM /Control_System/Closed Loop Control/FS-MPC 2 Vectores modulado Clean Power ==
  settings: updateMethod=DISCRETE
  data: I input; Gate output size=3; FEM input size=2; Pref input; Qref input; mode input; Ts parameter; R parameter; Ls parameter; ud parameter; gmax parameter; dyV parameter; Tab parameter

function Gate       = fcn(I,FEM,Pref,Qref,mode,Ts, R, Ls, ud, gmax,dyV, Tab)


%%%%%Init Parameters%%%%%%%

% Ts=single(2.5e-5);
% R=single(1) ;
%  L=single(2.02e-3);
%  M=(3/7)*L;
% %Lt=(7/3)*M;
% Ls=single(L+M);
% ud=single(170);
% gmax=single(1000);
n=single(15);

% Div=single(4); %%%%Numero de divisiones 
% dy0=single(0.12);
% dyV=(1-dy0);


%Tp=single(Ts*0.9);
 persistent    Gop jop Gates iApred iBpred  uApred uBpred status1 %tick status1 
     if isempty(Gates)
        Gates=single([0,0,0]');
        Gop=gmax;
        jop=single(1);
        iApred=single(0);
        iBpred=single(0);
        uApred=single(0);
        uBpred=single(0);
  
     end


%%%%%%Read mesurments%%%%%%%%%%%%
iA=I(1);
iB=I(2);
eA=FEM(1);
eB=FEM(2);
moder=mode;

% % 
% % indexv=[1,1,1,1,1,1,1,1,1,1,2,2,2,2,3;
% %         1,1,1,1,1,1,2,2,2,3,2,2,2,3,3;
% %         1,1,1,2,2,3,2,2,3,3,2,2,3,3,3;
% %         1,2,3,2,3,3,2,3,3,3,2,3,3,3,3;];

% Tab=[0 0;
%     0.25 0;
%     0 0.25;
%     0.5 0;
%     0.25 0.25
%     0 0.5;
%     0.75 0;
%     0.5 0.25;
%     0.25 0.5;
%     0 0.75;
%     1 0;
%     0.75 0.25
%     0.5 0.5
%     0.25 0.75
%     0 1];

if mode==1
   u1=ud*[0	,	0	;
2/3	,	0	;
1/3	,	1/sqrt(3)];
elseif mode==2
   u1=ud*[0	,	0	;
1/3	,	1/sqrt(3)	;
-1/3	,	1/sqrt(3)	;];   
elseif mode==3
   u1=ud*[0	,	0	;
-1/3	,	1/sqrt(3)	;
-2/3	,	0	;];  
 elseif mode==4
   u1=ud*[0	,	0	;
-2/3	,	0	;
-1/3	,	-1/sqrt(3)	;];
 elseif mode==5
   u1=ud*[0	,	0	;
-1/3	,	-1/sqrt(3)	;
1/3	,	-1/sqrt(3)	;];
 elseif mode==6
  u1=ud*[0	,	0	;
1/3	,	-1/sqrt(3)	;
2/3	,	0	;];
else
  u1=ud*[0	,	0	;
2/3	,	0	;
1/3	,	1/sqrt(3)]; 
end

%%%%%%%%FSMPC%%%%%%%%%%%%%%%%%%%%%%%%%%%%%%%%%%%%%

     Gop=gmax;
     jop=single(1);
     uA1=u1(2,1);
     uB1=u1(2,2);
     uA2=u1(3,1);
     uB2=u1(3,2);
%      P=iA*eA+iB*eB;
%      Q=iA*eB-iB*eA;
%%%%%%For n loop  %%%%%% 
     for j= 1:n    
   
    T1=Tab(j,1);
    T2=Tab(j,2);
    uA=dyV*(T1*uA1 + T2*uA2);%+dy0*uAnull;
    uB=dyV*(T1*uB1 + T2*uB2);%+dy0*uAnull;

%%%%%%For loop 3 combinacion de vectores%%%%%% 

     iA1= iA + (1/Ls)*(Ts*uA)- (Ts/Ls)*(eA+R*iA);
     iB1=iB + (1/Ls)*(Ts*uB)- (Ts/Ls)*(eB+R*iB);
%      P1=-P+iA1*eA+iB1*eB+iA*eA+iB*eB;
%      Q1=-Q+iA1*eB-iB1*eA+iA*eB-iB*eA;
    P1=iA1*eA+iB1*eB;
    Q1=iA1*eB-iB1*eA;

   %  G=(iAref-iA1)^2+(iBref-iB1)^2 ; 
      G=(Pref-P1)^2+(Qref-Q1)^2 ; 
          if G<Gop
          Gop=G;
          jop=j;
          
          end
     end
%%%%Apply conmutation states%%%%%%%%%%%%%%%%%%%%%%%  
Ta=dyV*Tab(jop,1);
Tb=dyV*Tab(jop,2);

TA=(moder==1)*(Tb+Ta)+(moder==6)*(Tb+Ta)+(moder==2)*(Ta)+(moder==5)*(Tb);
TB=(moder==1)*(Tb)+(moder==2)*(Tb+Ta)+(moder==3)*(Tb+Ta)+(moder==4)*(Ta);
TC=(moder==6)*(Ta)+(moder==3)*(Tb)+(moder==4)*(Tb+Ta)+(moder==5)*(Tb+Ta);
  

Gates=[TA,TB,TC]';
Gate=Gates;

== matlab function MicroFSMPCCLACPU1/ADC-PWM /Control_System/Closed Loop Control/FS-MPC 2 Vectores modulado Clean1 ==
  settings: updateMethod=DISCRETE
  data: I input; Gate output size=3; FEM input size=2; iAref input size=1; iBref input size=1; mode input; Ts parameter; R parameter; gmax parameter; dyV parameter; Tab parameter; ud parameter; Ls parameter

function Gate       = fcn(I,FEM,iAref,iBref,mode,Ts, R, gmax,dyV, Tab, ud, Ls)


%%%%%Init Parameters%%%%%%%

% Ts=single(2.5e-5);
% R=single(1) ;
%  L=single(2.02e-3);
%  M=(3/7)*L;
% %Lt=(7/3)*M;
% Ls=single(L+M);
% ud=single(170);
% gmax=single(1000);
n=single(15);

% Div=single(4); %%%%Numero de divisiones 
% dy0=single(0.12);
% dyV=(1-dy0);


%Tp=single(Ts*0.9);
 persistent    Gop jop Gates iApred iBpred  uApred uBpred status1 %tick status1 
     if isempty(Gates)
        Gates=single([0,0,0]');
        Gop=gmax;
        jop=single(1);
        iApred=single(0);
        iBpred=single(0);
        uApred=single(0);
        uBpred=single(0);
  
     end


%%%%%%Read mesurments%%%%%%%%%%%%
iA=I(1);
iB=I(2);
eA=FEM(1);
eB=FEM(2);
moder=mode;

% % 
% % indexv=[1,1,1,1,1,1,1,1,1,1,2,2,2,2,3;
% %         1,1,1,1,1,1,2,2,2,3,2,2,2,3,3;
% %         1,1,1,2,2,3,2,2,3,3,2,2,3,3,3;
% %         1,2,3,2,3,3,2,3,3,3,2,3,3,3,3;];

% Tab=[0 0;
%     0.25 0;
%     0 0.25;
%     0.5 0;
%     0.25 0.25
%     0 0.5;
%     0.75 0;
%     0.5 0.25;
%     0.25 0.5;
%     0 0.75;
%     1 0;
%     0.75 0.25
%     0.5 0.5
%     0.25 0.75
%     0 1];

if mode==1
   u1=ud*[0	,	0	;
2/3	,	0	;
1/3	,	1/sqrt(3)];
elseif mode==2
   u1=ud*[0	,	0	;
1/3	,	1/sqrt(3)	;
-1/3	,	1/sqrt(3)	;];   
elseif mode==3
   u1=ud*[0	,	0	;
-1/3	,	1/sqrt(3)	;
-2/3	,	0	;];  
 elseif mode==4
   u1=ud*[0	,	0	;
-2/3	,	0	;
-1/3	,	-1/sqrt(3)	;];
 elseif mode==5
   u1=ud*[0	,	0	;
-1/3	,	-1/sqrt(3)	;
1/3	,	-1/sqrt(3)	;];
 elseif mode==6
  u1=ud*[0	,	0	;
1/3	,	-1/sqrt(3)	;
2/3	,	0	;];
else
  u1=ud*[0	,	0	;
2/3	,	0	;
1/3	,	1/sqrt(3)]; 
end

%%%%%%%%FSMPC%%%%%%%%%%%%%%%%%%%%%%%%%%%%%%%%%%%%%

     Gop=gmax;
     jop=single(1);
     uA1=u1(2,1);
     uB1=u1(2,2);
     uA2=u1(3,1);
     uB2=u1(3,2);

%%%%%%For n loop  %%%%%% 
     for j= 1:n    
   
    T1=Tab(j,1);
    T2=Tab(j,2);
    uA=dyV*(T1*uA1 + T2*uA2);%+dy0*uAnull;
    uB=dyV*(T1*uB1 + T2*uB2);%+dy0*uAnull;

%%%%%%For loop 3 combinacion de vectores%%%%%% 

     iA1= iA + (1/Ls)*(Ts*uA)- (Ts/Ls)*(eA+R*iA);
     iB1=iB + (1/Ls)*(Ts*uB)- (Ts/Ls)*(eB+R*iB);
     
     G=(iAref-iA1)^2+(iBref-iB1)^2 ; 

          if G<Gop
          Gop=G;
          jop=j;
          
          end
     end
%%%%Apply conmutation states%%%%%%%%%%%%%%%%%%%%%%%  
Ta=dyV*Tab(jop,1);
Tb=dyV*Tab(jop,2);

TA=(moder==1)*(Tb+Ta)+(moder==6)*(Tb+Ta)+(moder==2)*(Ta)+(moder==5)*(Tb);
TB=(moder==1)*(Tb)+(moder==2)*(Tb+Ta)+(moder==3)*(Tb+Ta)+(moder==4)*(Ta);
TC=(moder==6)*(Ta)+(moder==3)*(Tb)+(moder==4)*(Tb+Ta)+(moder==5)*(Tb+Ta);
  

Gates=[TA,TB,TC]';
Gate=Gates;

== matlab function MicroFSMPCCLACPU1/ADC-PWM /Control_System/Closed Loop Control/FS-MPC 2 Vectores modulado1 ==
  settings: updateMethod=DISCRETE
  data: I input; Gate output size=3; FEM input size=2; iAref input; iBref input; mode input; Vbus input

function Gate       = fcn(I,FEM,iAref,iBref,mode,Vbus)


%%%%%Init Parameters%%%%%%%
%Ts=single(5e-5);
Ts=single(3.2e-05);
R=single(1) ;
%L=single(9.75e-3);
 L=single(2.02e-3);
 M=(3/7)*L;
%Lt=(7/3)*M;
Ls=single(L+M);
%Ls=single(L);
%Ls=single(L);
%ud=240;
%ud=single(Vbus);
ud=single(170);
%Kt =single(0.3811);
%T0=Ts*(1);
%Ke=single(0.3455);
gmax=single(1000);
n=single(15);

% uAnull=single(0);
% uBnull=single(0);
Div=single(4); %%%%Numero de divisiones 
dy0=single(0.12);
dyV=(1-dy0)/Div;


%Tp=single(Ts*0.9);
 persistent    Gop jop Gates iApred iBpred  uApred uBpred status1 %tick status1 
     if isempty(Gates)
        Gates=single([0,0,0]');
        Gop=gmax;
        jop=single(1);
        iApred=single(0);
        iBpred=single(0);
        uApred=single(0);
        uBpred=single(0);
  
     end


%%%%%%Read mesurments%%%%%%%%%%%%
iA=I(1);
iB=I(2);
eA=FEM(1);
eB=FEM(2);
moder=mode;
% eA1=FEM1(1);
% eB1=FEM1(2);
% fa=eA/(Ke*w);
% fb=eB/(Ke*w);
% fa1=fa;
% fb1=fb;
% ua=u(1);
% ub=u(2);



 % % %%%7 vectores ordenados ab separados flotando
%  status1=[0,1,0,1,0,1	;
%      1,0,0,0,0,1	;
%  0,0,1,0,0,1	;
%  0,1,1,0,0,0	;
%  0,1,0,0,1,0	;
%  0,0,0,1,1,0	;
%  1,0,0,1,0,0	;];
% 
%  u1=ud*[0	,	0	;
%      1/2	,	sqrt(3)/6 	;
% 0	,	sqrt(3)/3	;
% -1/2	,	sqrt(3)/6 	;
% -1/2	,	-sqrt(3)/6 	;
% 0	,	-sqrt(3)/3	;
% 1/2	,	-sqrt(3)/6 	;
% ];

%%%%%%For loop 3%%%%%%      
% %%%7 vectores ordenados ab tradicionales
%  status1=[1,1,1;
%           1,0,0	;
%           1,1,0;
%           0,1,0;
%            0,1,1	;
%            0,0,1	;
%            1,0,1;
%            ];
% % 
%  u1=ud*[0	,	0	;
%       2/3	,	0	;
%       1/3	,	1/sqrt(3)	;%parece estar aml el vector
%   -1/3	,	1/sqrt(3)	;
%  -2/3	,	0	;
%  -1/3	,	-1/sqrt(3)	;
%   1/3	,	-1/sqrt(3)	;
%   ];
indexv=[1,1,1,1,1,1,1,1,1,1,2,2,2,2,3;
        1,1,1,1,1,1,2,2,2,3,2,2,2,3,3;
        1,1,1,2,2,3,2,2,3,3,2,2,3,3,3;
        1,2,3,2,3,3,2,3,3,3,2,3,3,3,3;];
%%%%%Modos 2 vectores con VO
% if mode==1
%  status1=[0,0,0;
% 1,1,0	;
% 0,1,0	;];   
%  u1=ud*[0	,	0	;
% 1/3	,	1/sqrt(3)	;
% -1/3	,	1/sqrt(3)	;];   
% elseif mode==2
%  status1=[0,0,0;
% 0,1,0	;
% 0,1,1	;];   
%  u1=ud*[0	,	0	;
% -1/3	,	1/sqrt(3)	;
% -2/3	,	0	;];  
%  elseif mode==3
%  status1=[0,0,0;
%  0,1,1	;
% 0,0,1	;];   
%  u1=ud*[0	,	0	;
% -2/3	,	0	;
% -1/3	,	-1/sqrt(3)	;];
%  elseif mode==4
%  status1=[0,0,0;
%  0,0,1	;
% 1,0,1	;];   
%  u1=ud*[0	,	0	;
% -1/3	,	-1/sqrt(3)	;
% 1/3	,	-1/sqrt(3)	;];
%  elseif mode==5
%  status1=[0,0,0
% 1,0,1	;
%  1,0,0	;];   
%  u1=ud*[0	,	0	;
% 1/3	,	-1/sqrt(3)	;
% 2/3	,	0	;];
%  elseif mode==6
%  status1=[0,0,0;
%  1,0,0	;
% 1,1,0;];   
%  u1=ud*[0	,	0	;
% 2/3	,	0	;
% 1/3	,	1/3	;];
% else
%    status1=[0,0,0;
% 1,1,0	;
% 0,1,0	;];   
%  u1=ud*[0	,	0	;
% 1/3	,	1/sqrt(3)	;
% -1/3	,	1/sqrt(3)	;]; 
% end

%Vpred=[uApred;uBpred];

 if mode==1
  
 u1=ud*[0	,	0	;
2/3	,	0	;
1/3	,	1/sqrt(3)];
elseif mode==2
  
 u1=ud*[0	,	0	;
1/3	,	1/sqrt(3)	;
-1/3	,	1/sqrt(3)	;];   
elseif mode==3
  
 u1=ud*[0	,	0	;
-1/3	,	1/sqrt(3)	;
-2/3	,	0	;];  
 elseif mode==4
  
 u1=ud*[0	,	0	;
-2/3	,	0	;
-1/3	,	-1/sqrt(3)	;];
 elseif mode==5
   
 u1=ud*[0	,	0	;
-1/3	,	-1/sqrt(3)	;
1/3	,	-1/sqrt(3)	;];
 elseif mode==6
  
 u1=ud*[0	,	0	;
1/3	,	-1/sqrt(3)	;
2/3	,	0	;];

else
  
 u1=ud*[0	,	0	;
2/3	,	0	;
1/3	,	1/sqrt(3)]; 
end

%%%%%%%%FSMPC%%%%%%%%%%%%%%%%%%%%%%%%%%%%%%%%%%%%%

     Gop=gmax;
      jop=single(1);

%%%%%%For n loop  %%%%%% 
     for j= 1:n    
     uA1=u1(indexv(1,j),1);
     uB1=u1(indexv(1,j),2);
     uA2=u1(indexv(2,j),1);
     uB2=u1(indexv(2,j),2);
     uA3=u1(indexv(3,j),1);
     uB3=u1(indexv(3,j),2);
     uA4=u1(indexv(4,j),1);
     uB4=u1(indexv(4,j),2);

%%%%%%For loop 3 combinacion de vectores%%%%%% 

       uA=dyV*(uA1 + uA2+ uA3 + uA4);%+dy0*uAnull;
       uB=dyV*(uB1 + uB2+ uB3 + uB4);%+dy0*uAnull;


     iA1= iA + (1/Ls)*(Ts*uA)- (Ts/Ls)*(eA+R*iA);
     iB1=iB + (1/Ls)*(Ts*uB)- (Ts/Ls)*(eB+R*iB);
     
     G=(iAref-iA1)^2+(iBref-iB1)^2 ; 

          if G<Gop
          Gop=G;
          jop=j;
          iApred=iA1;
          iBpred=iB1;
   
          end
     end

    
%%%%Apply conmutation states%%%%%%%%%%%%%%%%%%%%%%%  


   % Gates=status1(jop,:)';

%To=dyV*((indexv(1,jop)==1)+(indexv(2,jop)==1)+(indexv(3,jop)==1)+(indexv(4,jop)==1))+dy0;
To=0;
Ta=dyV*((indexv(1,jop)==2)+(indexv(2,jop)==2)+(indexv(3,jop)==2)+(indexv(4,jop)==2));
Tb=dyV*((indexv(1,jop)==3)+(indexv(2,jop)==3)+(indexv(3,jop)==3)+(indexv(4,jop)==3));


  TA=(moder==1)*(Tb+Ta)+(moder==6)*(Tb+Ta)+(moder==2)*(Ta)+(moder==5)*(Tb);
  TB=(moder==1)*(Tb)+(moder==2)*(Tb+Ta)+(moder==3)*(Tb+Ta)+(moder==4)*(Ta);
  TC=(moder==6)*(Ta)+(moder==3)*(Tb)+(moder==4)*(Tb+Ta)+(moder==5)*(Tb+Ta);

% TA=(moder==6)*(To+Tb+Ta)+(moder==5)*(To+Tb+Ta)+(moder==1)*(To+Ta)+(moder==2)*(To)+(moder==3)*(To)+(moder==4)*(To+Tb);
% TB=(moder==5)*(To)+(moder==6)*(To+Tb)+(moder==1)*(To+Tb+Ta)+(moder==2)*(To+Tb+Ta)+(moder==3)*(To+Ta)+(moder==4)*(To);
% TC=(moder==5)*(To+Ta)+(moder==6)*(To)+(moder==1)*(To)+(moder==2)*(To+Tb)+(moder==3)*(To+Tb+Ta)+(moder==4)*(To+Tb+Ta);

Gates=[TA,TB,TC]';
% J=jop;
 Gate=Gates;
% Ipred=[iApred;iBpred];
%tie=t2;
%jl=jn;
%j=1;




%   TA=(moder==1)*(To+Tb+Ta)+(moder==6)*(To+Tb+Ta)+(moder==2)*(To+Ta)+(moder==3)*(To)+(moder==4)*(To)+(moder==5)*(To+Tb);
% % TA=(moder==6)*(To+Tb+Ta)+(moder==5)*(To+Tb+Ta)+(moder==1)*(To+Ta)+(moder==2)*(To)+(moder==3)*(To)+(moder==4)*(To+Tb);
%   TB=(moder==6)*(To)+(moder==1)*(To+Tb)+(moder==2)*(To+Tb+Ta)+(moder==3)*(To+Tb+Ta)+(moder==4)*(To+Ta)+(moder==5)*(To);
% % TB=(moder==5)*(To)+(moder==6)*(To+Tb)+(moder==1)*(To+Tb+Ta)+(moder==2)*(To+Tb+Ta)+(moder==3)*(To+Ta)+(moder==4)*(To);
%   TC=(moder==6)*(To+Ta)+(moder==1)*(To)+(moder==2)*(To)+(moder==3)*(To+Tb)+(moder==4)*(To+Tb+Ta)+(moder==5)*(To+Tb+Ta);

== matlab function MicroFSMPCCLACPU1/ADC-PWM /Control_System/Closed Loop Control/FS-MPC 2 Vectores simple1 ==
  settings: updateMethod=DISCRETE
  data: I input; Gate output size=3; FEM input; iAref input; iBref input; J output size=1; mode input

function [Gate,J]      = fcn(I,FEM,iAref,iBref,mode)
%function [Gate,J,Vpred,Ipred]      = fcn(I,FEM,iAref,iBref,Vbus,mode)


%%%%%Init Parameters%%%%%%%
Ts=single(3.2e-5);
%Ts=single(3.2e-05);
%Ts=single(3.125e-05);
R=single(1) ;
%L=single(4.75e-3);
%L=single(1.4e-3);
L=single(1.4e-3);
%L=single(2.02e-3);
%L=single(Lp);
M=(3/7)*L;
%Lt=(7/3)*M;
Ls=single(L+M);
%Ls=single(L);
ud=single(170);
%ud=single(Vbus);
%T0=Ts*(1);
gmax=single(10000);
n=single(3);
Tp=single(Ts*0.9);
uAnull=single(0);
uBnull=single(0);
%b=0.4;
 persistent    Gop jop Gates iApred iBpred blk %status1 %tick status1 
     if isempty(Gates)
        Gates=[0,0,0]';
        Gop=gmax;
        jop=single(1);
         iApred=single(0);
         iBpred=single(0);
          blk=single(0);
%        status1=[0,0,0;
% 1,1,0;
% 0,1,0;]; 
     end


%%%%%%Read mesurments%%%%%%%%%%%%
iA=I(1);
iB=I(2);
eA=FEM(1);
eB=FEM(2);
% eA1=FEM1(1);
% eB1=FEM1(2);
% fa=eA/(Ke*w);
% fb=eB/(Ke*w);
% fa1=fa;
% fb1=fb;
% ua=u(1);
% ub=u(2);



 % % %%%7 vectores ordenados ab separados flotando
%  status1=[0,1,0,1,0,1	;
%      1,0,0,0,0,1	;
%  0,0,1,0,0,1	;
%  0,1,1,0,0,0	;
%  0,1,0,0,1,0	;
%  0,0,0,1,1,0	;
%  1,0,0,1,0,0	;];
% 
%  u1=ud*[0	,	0	;
%      1/2	,	sqrt(3)/6 	;
% 0	,	sqrt(3)/3	;
% -1/2	,	sqrt(3)/6 	;
% -1/2	,	-sqrt(3)/6 	;
% 0	,	-sqrt(3)/3	;
% 1/2	,	-sqrt(3)/6 	;
% ];

%%%%%%For loop 3%%%%%%      
% %%%7 vectores ordenados ab tradicionales
%  status1= [0,0,0;
%            1,0,0	;
%            1,1,0;
%            0,1,0;
%            0,1,1	;
%            0,0,1	;
%            1,0,1; ];
% % 
%  u1=ud*[0	,	0	;
%       2/3	,	0	;
%       1/3	,	1/sqrt(3)	;%parece estar aml el vector
%   -1/3	,	1/sqrt(3)	;
%  -2/3	,	0	;
%  -1/3	,	-1/sqrt(3)	;
%   1/3	,	-1/sqrt(3)	;
%   ];

%%%%%Modos 2 vectores con VO
% if mode==1
%  status1=[0,0,0;
% 1,1,0	;
% 0,1,0	;];   
%  u1=ud*[0	,	0	;
% 1/3	,	1/sqrt(3)	;
% -1/3	,	1/sqrt(3)	;];   
% elseif mode==2
%  status1=[0,0,0;
% 0,1,0	;
% 0,1,1	;];   
%  u1=ud*[0	,	0	;
% -1/3	,	1/sqrt(3)	;
% -2/3	,	0	;];  
%  elseif mode==3
%  status1=[0,0,0;
%  0,1,1	;
% 0,0,1	;];   
%  u1=ud*[0	,	0	;
% -2/3	,	0	;
% -1/3	,	-1/sqrt(3)	;];
%  elseif mode==4
%  status1=[0,0,0;
%  0,0,1	;
% 1,0,1	;];   
%  u1=ud*[0	,	0	;
% -1/3	,	-1/sqrt(3)	;
% 1/3	,	-1/sqrt(3)	;];
%  elseif mode==5
%  status1=[0,0,0
% 1,0,1	;
%  1,0,0	;];   
%  u1=ud*[0	,	0	;
% 1/3	,	-1/sqrt(3)	;
% 2/3	,	0	;];
%  elseif mode==6
%  status1=[0,0,0;
%  1,0,0	;
% 1,1,0;];   
%  u1=ud*[0	,	0	;
% 2/3	,	0	;
% 1/3	,	1/3	;];
% else
%    status1=[0,0,0;
% 1,1,0	;
% 0,1,0	;];   
%  u1=ud*[0	,	0	;
% 1/3	,	1/sqrt(3)	;
% -1/3	,	1/sqrt(3)	;]; 
% end

%%%%% Como en sim 
 if mode==1
 status1=[0,0,0;
 1,0,0	;
1,1,0;];   
 u1=ud*[0	,	0	;
2/3	,	0	;
1/3	,	1/sqrt(3)];
elseif mode==2
 status1=[0,0,0;
1,1,0	;
0,1,0	;];   
 u1=ud*[0	,	0	;
1/3	,	1/sqrt(3)	;
-1/3	,	1/sqrt(3)	;];   
elseif mode==3
 status1=[0,0,0;
0,1,0	;
0,1,1	;];   
 u1=ud*[0	,	0	;
-1/3	,	1/sqrt(3)	;
-2/3	,	0	;];  
 elseif mode==4
 status1=[0,0,0;
 0,1,1	;
0,0,1	;];   
 u1=ud*[0	,	0	;
-2/3	,	0	;
-1/3	,	-1/sqrt(3)	;];
 elseif mode==5
 status1=[0,0,0;
 0,0,1	;
1,0,1	;];   
 u1=ud*[0	,	0	;
-1/3	,	-1/sqrt(3)	;
1/3	,	-1/sqrt(3)	;];
 elseif mode==6
 status1=[0,0,0
1,0,1	;
 1,0,0	;];   
 u1=ud*[0	,	0	;
1/3	,	-1/sqrt(3)	;
2/3	,	0	;];

else
 status1=[0,0,0;
 1,0,0	;
1,1,0;];   
 u1=ud*[0	,	0	;
2/3	,	0	;
1/3	,	1/sqrt(3)]; 
end


%%%%%nurva


%  if mode==1
%  status1=[0,0,0;
%  1,0,0	;
% 1,1,0;];   
%  u1=ud*[0	,	0	;
% 2/3	,	0	;
% 1/3	,	1/sqrt(3)];
% elseif mode==2
%  status1=[0,0,0;
% 1,1,0	;
% 0,1,0	;];   
%  u1=ud*[0	,	0	;
% 1/3	,	1/sqrt(3)	;
% -1/3	,	1/sqrt(3)	;];   
% elseif mode==3
%  status1=[0,0,0;
% 0,1,0	;
% 0,1,1	;];   
%  u1=ud*[0	,	0	;
% -1/3	,	1/sqrt(3)	;
% -2/3	,	0	;];  
%  elseif mode==4
%  status1=[0,0,0;
%  0,1,1	;
% 0,0,1	;];   
%  u1=ud*[0	,	0	;
% -2/3	,	0	;
% -1/3	,	-1/sqrt(3)	;];
%  elseif mode==5
%  status1=[0,0,0;
%  0,0,1	;
% 1,0,1	;];   
%  u1=ud*[0	,	0	;
% -1/3	,	-1/sqrt(3)	;
% 1/3	,	-1/sqrt(3)	;];
%  elseif mode==6
%  status1=[0,0,0
% 1,0,1	;
%  1,0,0	;];   
%  u1=ud*[0	,	0	;
% 1/3	,	-1/sqrt(3)	;
% 2/3	,	0	;];
% 
% else
%  status1=[0,0,0;
%  1,0,0	;
% 1,1,0;];   
%  u1=ud*[0	,	0	;
% 2/3	,	0	;
% 1/3	,	1/sqrt(3)]; 
% end



%%%%%%%%FSMPC%%%%%%%%%%%%%%%%%%%%%%%%%%%%%%%%%%%%%

     Gop=gmax;
     % jop=single(1);

%%%%%%For n loop  %%%%%% 
     for j= 1:n    
     uA1=u1(j,1);
     uB1=u1(j,2);
%      S1=status1(j,1);
%      S2=status1(j,2);
%      S3=status1(j,3);

     iA1= iA + (1/Ls)*(Tp*uA1)- (Ts/Ls)*(eA+R*iA);
     iB1=iB + (1/Ls)*(Tp*uB1)- (Ts/Ls)*(eB+R*iB);
     
     %Z=(S1-Gates(1))^2+(S2-Gates(2))^2+(S3-Gates(3))^2;
     
     G=(iAref-iA1)^2+(iBref-iB1)^2;%+ b*Z ; 

          if G<Gop
          Gop=G;
          jop=j;
          iApred=iA1;
           iBpred=iB1;
          end
     end

    
%%%%Apply conmutation states%%%%%%%%%%%%%%%%%%%%%%%  
% if blk>0.5
% blk=single(0);
% else
% blk=blk+single(1);
% end
% beat=blk;



Gates=status1(jop,:)';
% UA=Tp/Ts*u1(jop,1) ;%+(Ts-Tp)/Ts*uAnull;
% UB=Tp/Ts*u1(jop,2) ;%+(Ts-Tp)/Ts*uBnull;
%Gates=status1(jop,:)';
J=jop;
Gate=Gates;
% Vpred=[UA;UB];
%  Ipred=[iApred;iBpred];
%tie=t2;
%jl=jn;
%j=1;

== matlab function MicroFSMPCCLACPU1/ADC-PWM /Control_System/Closed Loop Control/FS-MPC 2 Vectores simple2 ==
  settings: updateMethod=DISCRETE
  data: I input; FEM input; U input; Ipred output

function Ipred       = fcn(I,FEM,U)


%%%%%Init Parameters%%%%%%%
Ts=single(5e-5);
R=single(1.2) ;
L=single(4.75e-3);
% M=L;
% Lt=(7/3)*M;
% Ls=single(Lt+M);
%ud=240;




%%%%%%Read mesurments%%%%%%%%%%%%
iA=I(1);
iB=I(2);
eA=FEM(1);
eB=FEM(2);
uA1=U(1);
uB1=U(2);

 

L=Ts(-R*iA+UA1+eA)/(iA-iA1)     
iA1= iA + (1/Ls)*(uA1*Ts)- (Ts/Ls)*(eA+R*iA);
     iB1=iB + (1/Ls)*(uB1*Ts)- (Ts/Ls)*(eB+R*iB);
     



Ipred=[iA1;iB1];

== matlab function MicroFSMPCCLACPU1/ADC-PWM /Control_System/Closed Loop Control/FS-MPC 2 Vectores simple3 ==
  settings: updateMethod=DISCRETE
  data: I input; FEM input; U input; L output

function L       = fcn(I,FEM,U)


%%%%%Init Parameters%%%%%%%
Ts=single(5e-5);
R=single(1.2) ;
%L=single(4.75e-3);
% M=L;
% Lt=(7/3)*M;
% Ls=single(Lt+M);
%ud=240;

 persistent    iA1
     if isempty(iA1)
iA1=single(0); 
     end


%%%%%%Read mesurments%%%%%%%%%%%%
iA=I(1);
iB=I(2);
eA=FEM(1);
eB=FEM(2);
uA1=U(1);
uB1=U(2);

 

Ls=Ts(-R*iA+UA1+eA)/(iA-iA1);

iA1= iA;
     



L=Ls;
